simulink model "Helicopter_Kalman_filter"  (R2018a)
settings: Solver=VariableStepAuto  StartTime=0.0  StopTime=inf  RelTol=1e-3
values from neighbouring files (symbols this model uses):
  Ad = sys_d.a    [Helicopter_Values.m]
  Bd = sys_d.b    [Helicopter_Values.m]
  Bp = 0.01    [Helicopter_Values.m]
  By = 0.08    [Helicopter_Values.m]
  Cd = sys_d.c    [Helicopter_Values.m]
  g = 9.81    [Helicopter_Values.m]
  jeqp = 0.0172    [Helicopter_Values.m]
  jeqy = 0.021    [Helicopter_Values.m]
  kpp = 0.0556    [Helicopter_Values.m]
  kpy = 0.005    [Helicopter_Values.m]
  kyp = 0.15    [Helicopter_Values.m]
  kyy = 0.21084    [Helicopter_Values.m]
  lcm = 0.015    [Helicopter_Values.m]
  mheli = 0.479    [Helicopter_Values.m]
  p_r_op = -10*pi/180    (= -0.174532925199)    [Helicopter_Values.m]
  Vmp_op = (kyy*mheli*g*cos(p_r_op)*lcm)/(kyy*kpp -kyp*kpy)    [Helicopter_Values.m]
  Vmy_op = kyp*Vmp_op/kyy    [Helicopter_Values.m]
  wp_op = 0    [Helicopter_Values.m]
  wy_op = 0    [Helicopter_Values.m]
  y_r_op = pi/2    (= 1.57079632679)    [Helicopter_Values.m]
undefined symbols (not defined in the file or in its folder): K
libraries: realtime_pacer_lib x1
settings Model: Creator=pacoa  LastModifiedBy=pacoa

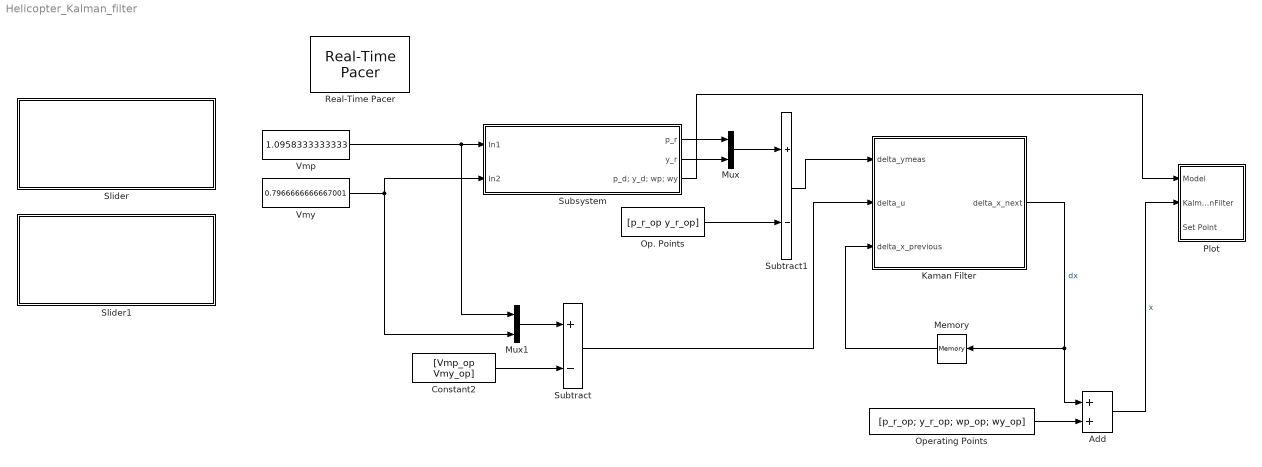
== system Helicopter_Kalman_filter ==
  Add : Sum
  Constant2 : Constant  Value=[Vmp_op Vmy_op]
  Kaman Filter : MATLAB Function  TreatAsAtomicUnit=on
  Memory : Memory  InitialCondition=[0;0;0;0]
  Mux : Mux  Inputs=2
  Mux1 : Mux  Inputs=2
  Op. Points : Constant  Value=[p_r_op y_r_op]
  Operating Points : Constant  Value=[p_r_op; y_r_op; wp_op; wy_op]
  Plot : Subsystem
  Real-Time Pacer : realtime_pacer_lib/Real-Time Pacer  simTimePerRealTime=1
  Slider : Subsystem  DialogController=hmiCreateDDGDialog  IsWebBlock=on  mask(MWDashboardBlock){webBlockId=04463d73-d6a9-4b3d-abfe-2f563ab264e6, webBlockType=slider, ShowInLibBrowser=on, ShowInitialText=on, HMISrcModelName=Helicopter_Kalman_filter}
      mask prompts: webBlockId "WebBlock Id"; webBlockType "WebBlock Type"; HMISrcModelName "Source Model"
      mask help: SimulinkHMI:dialogs:SliderDialogDesc
      mask Help: helpview([docroot '/mapfiles/simulink.map'], 'hmi_slider')
      mask Display:
      | if strcmp(get_param(bdroot(gcb),'BlockDiagramType'), 'library')
      |     image([(matlabroot) '/toolbox/simulink/hmi/icons/Slider.png']);
      | end
  Slider1 : Subsystem  DialogController=hmiCreateDDGDialog  IsWebBlock=on  mask(MWDashboardBlock){webBlockId=82fec370-2a65-419d-b4f2-61c4ae5ab55a, webBlockType=slider, ShowInLibBrowser=on, ShowInitialText=on, HMISrcModelName=Helicopter_Kalman_filter}
      mask prompts: webBlockId "WebBlock Id"; webBlockType "WebBlock Type"; HMISrcModelName "Source Model"
      mask help: SimulinkHMI:dialogs:SliderDialogDesc
      mask Help: helpview([docroot '/mapfiles/simulink.map'], 'hmi_slider')
      mask Display:
      | if strcmp(get_param(bdroot(gcb),'BlockDiagramType'), 'library')
      |     image([(matlabroot) '/toolbox/simulink/hmi/icons/Slider.png']);
      | end
  Subsystem : Subsystem
  Subtract : Sum  Inputs=+-
  Subtract1 : Sum  Inputs=+-
  Vmp : Constant  Value=1.0958333333333
  Vmy : Constant  Value=0.7966666666667001
  wires:
  Vmp/1 -> Mux1/1, Subsystem/1(In1)
  Vmy/1 -> Subsystem/2(In2), Mux1/2
  Subsystem/1(p_r) -> Mux/1
  Subsystem/2(y_r) -> Mux/2
  Memory/1 -> Kaman Filter/3(delta_x_previous)
  Mux1/1 -> Subtract/1
  Constant2/1 -> Subtract/2
  Mux/1 -> Subtract1/1
  Op. Points/1 -> Subtract1/2
  Subtract/1 -> Kaman Filter/2(delta_u)
  Subtract1/1 -> Kaman Filter/1(delta_ymeas)
  Subsystem/3(p_d; y_d; wp; wy) -> Plot/1(Model)
  Kaman Filter/1(delta_x_next) -> Memory/1, Add/1  "dx"
  Operating Points/1 -> Add/2
  Add/1 -> Plot/2(KalmanFilter)  "x"

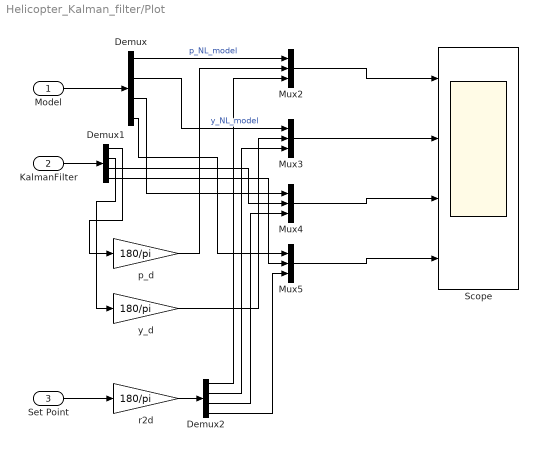
== system Helicopter_Kalman_filter/Plot ==
  Model : Inport
  KalmanFilter : Inport  Port=2
  Set Point : Inport  Port=3
  Demux : Demux
  Demux1 : Demux
  Demux2 : Demux
  Mux{2..5} (4 alike) : Mux  Inputs=3
  Scope : Scope  NumInputPorts=4
  p_d : Gain  Gain=180/pi
  r2d : Gain  Gain=180/pi
  y_d : Gain  Gain=180/pi
  wires:
  KalmanFilter/1 -> Demux1/1
  Mux2/1 -> Scope/1
  Demux/3 -> Mux4/1
  Demux1/4 -> Mux5/2
  Mux4/1 -> Scope/3
  Demux1/3 -> Mux4/2
  Demux/1 -> Mux2/1  "p_NL_model"
  Demux/4 -> Mux5/1
  Mux3/1 -> Scope/2
  p_d/1 -> Mux2/2
  Mux5/1 -> Scope/4
  Demux1/1 -> p_d/1
  y_d/1 -> Mux3/2
  Demux/2 -> Mux3/1  "y_NL_model"
  Demux1/2 -> y_d/1
  Model/1 -> Demux/1
  Set Point/1 -> r2d/1
  r2d/1 -> Demux2/1
  Demux2/1 -> Mux2/3
  Demux2/2 -> Mux3/3
  Demux2/3 -> Mux4/3
  Demux2/4 -> Mux5/3

== system Helicopter_Kalman_filter/Slider ==

== system Helicopter_Kalman_filter/Slider1 ==

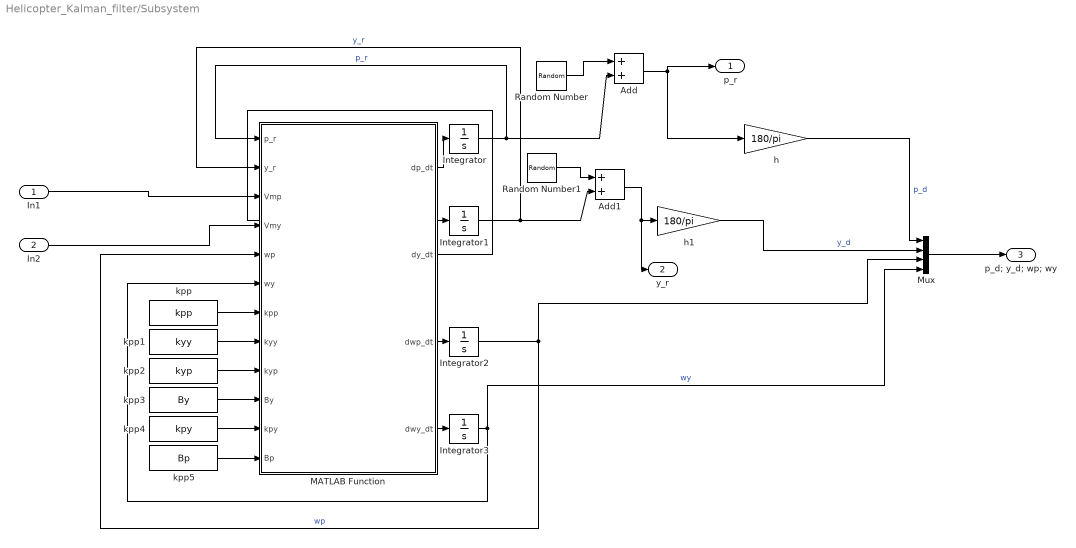
== system Helicopter_Kalman_filter/Subsystem ==
  In1 : Inport
  In2 : Inport  Port=2
  Add : Sum
  Add1 : Sum
  Integrator : Integrator  InitialCondition=(p_r_op)  LimitOutput=on  UpperSaturationLimit=pi/4  LowerSaturationLimit=-pi/4
  Integrator1 : Integrator  InitialCondition=(y_r_op)  LimitOutput=on  UpperSaturationLimit=pi  LowerSaturationLimit=0
  Integrator2 : Integrator  UpperSaturationLimit=1  LowerSaturationLimit=-1
  Integrator3 : Integrator
  MATLAB Function : MATLAB Function  TreatAsAtomicUnit=on
  Mux : Mux
  Random Number : RandomNumber  Variance=0.0005  SampleTime=0.1
  Random Number1 : RandomNumber  Variance=0.0005  SampleTime=0.1
  h : Gain  Gain=180/pi
  h1 : Gain  Gain=180/pi
  kpp : Constant  Value=kpp
  kpp1 : Constant  Value=kyy
  kpp2 : Constant  Value=kyp
  kpp3 : Constant  Value=By
  kpp4 : Constant  Value=kpy
  kpp5 : Constant  Value=Bp
  p_r : Outport
  y_r : Outport  Port=2
  p_d; y_d; wp; wy : Outport  Port=3
  wires:
  kpp/1 -> MATLAB Function/7(kpp)
  In2/1 -> MATLAB Function/4(Vmy)
  kpp2/1 -> MATLAB Function/9(kyp)
  kpp4/1 -> MATLAB Function/11(kpy)
  MATLAB Function/3(dwp_dt) -> Integrator2/1
  Integrator1/1 -> Add1/2, MATLAB Function/2(y_r)  "y_r"
  Integrator3/1 -> Mux/4, MATLAB Function/6(wy)  "wy"
  MATLAB Function/1(dp_dt) -> Integrator/1
  h/1 -> Mux/1  "p_d"
  kpp3/1 -> MATLAB Function/10(By)
  kpp1/1 -> MATLAB Function/8(kyy)
  MATLAB Function/4(dwy_dt) -> Integrator3/1
  Integrator/1 -> Add/2, MATLAB Function/1(p_r)  "p_r"
  h1/1 -> Mux/2  "y_d"
  Integrator2/1 -> Mux/3, MATLAB Function/5(wp)  "wp"
  MATLAB Function/2(dy_dt) -> Integrator1/1
  kpp5/1 -> MATLAB Function/12(Bp)
  Mux/1 -> p_d; y_d; wp; wy/1
  In1/1 -> MATLAB Function/3(Vmp)
  Random Number/1 -> Add/1
  Add/1 -> h/1, p_r/1
  Random Number1/1 -> Add1/1
  Add1/1 -> y_r/1, h1/1

== matlab function Helicopter_Kalman_filter/Kaman Filter ==
  data: delta_ymeas input; delta_u input; delta_x_next output; delta_x_previous input size=[4; 1]; K parameter; Ad parameter; Bd parameter; Cd parameter
function delta_x_next = mykalman(delta_ymeas,delta_u,delta_x_previous, K, Ad, Bd, Cd)

delta_x_next = Ad*delta_x_previous +Bd*delta_u +K*(delta_ymeas -Cd*delta_x_previous);

== matlab function Helicopter_Kalman_filter/Subsystem/MATLAB Function ==
  data: p_r input; y_r input; Vmp input; Vmy input; wp input; dp_dt output size=[1 1]; wy input; dy_dt output size=[1 1]; dwp_dt output size=[1 1]; dwy_dt output size=[1 1]; lcm parameter; mheli parameter; jeqp parameter; jeqy parameter; g parameter; kpp input; kyy input; kyp input; By input; kpy input; Bp input
function [dp_dt, dy_dt, dwp_dt, dwy_dt]= fcn(p_r,y_r,Vmp, Vmy,wp,wy, lcm, mheli, jeqp, jeqy, g, kpp, kyy, kyp, By, kpy, Bp)

  %%Parameters
%   
%   Bp,
%   By,
%   g,
%   kpp,
%   kyp,
%   kyy,
%   kpy,
%   mheli,
%   lcm,
%   jeqp,
%   jeqy,
  

%%
   dp_dt = wp;
   dy_dt = wy;
   
   %%
   dwp_dt_n1 = (kpp*Vmp);
   dwp_dt_n2 = (kpy*Vmy);
   dwp_dt_n3 = (Bp*wp+ (mheli*(wy.^2)*sin(p_r)*(lcm^2)*cos(p_r) + (mheli*g*cos(p_r)*lcm)));
   
   dwp_dt_d = (jeqp + mheli*(lcm^2));
   
   dwp_dt = (dwp_dt_n1 -dwp_dt_n2 - dwp_dt_n3)/(dwp_dt_d);
   
   %%
   dwy_dt_n1 = kyp*Vmp;
   dwy_dt_n2 = kyy*Vmy;
   dwy_dt_n3 = 2*mheli*(wy)*sin(p_r)*(lcm^2)*cos(p_r)*wp;
   dwy_dt_n4 = By*wy;
   
   dwy_dt_d = jeqy + mheli*((cos(p_r))^2)*(lcm^2);
   
   dwy_dt = (dwy_dt_n1 - dwy_dt_n2 + dwy_dt_n3 -dwy_dt_n4)/(dwy_dt_d);
